simulink model "chutcalc_v2"  (R2019a)
settings: Solver=VariableStepDiscrete  StartTime=0.0  StopTime=10.0  RelTol=1e-3
undefined symbols (not defined in the file or in its folder): chutecalc_input
libraries: aerolibatmos2 x2
settings Model: Creator=onurd  LastModifiedBy=onurd

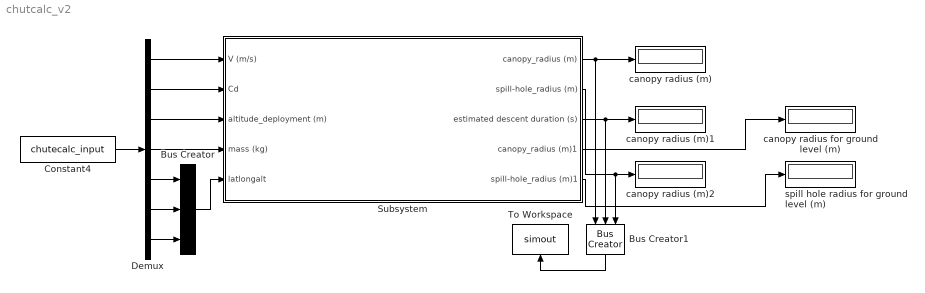
== system chutcalc_v2 ==
  " spill hole radius for ground level (m)" : Display
  Bus Creator : BusCreator  Inputs=3
  Bus Creator1 : BusCreator  Inputs=3
  Constant4 : Constant  Value=chutecalc_input
  Demux : Demux  Outputs=7
  Subsystem : Subsystem
  To Workspace : ToWorkspace  VariableName=simout  SampleTime=-1
      settings: MaxDataPoints=1  Save2DSignal=2-D array (concatenate along first dimension)
  canopy radius (m) : Display
  canopy radius (m)1 : Display
  canopy radius (m)2 : Display
  canopy radius for ground level (m) : Display
  wires:
  Subsystem/1(canopy_radius (m)) -> Bus Creator1/1, canopy radius (m)/1
  Constant4/1 -> Demux/1
  Demux/1 -> Subsystem/1(V (m/s))
  Demux/2 -> Subsystem/2(Cd)
  Demux/3 -> Subsystem/3(altitude_deployment (m))
  Demux/4 -> Subsystem/4(mass (kg))
  Demux/5 -> Bus Creator/1
  Demux/6 -> Bus Creator/2
  Demux/7 -> Bus Creator/3
  Bus Creator/1 -> Subsystem/5(latlongalt)
  Subsystem/2(spill-hole_radius (m)) -> canopy radius (m)1/1, Bus Creator1/2
  Subsystem/3(estimated descent duration (s)) -> canopy radius (m)2/1, Bus Creator1/3
  Bus Creator1/1 -> To Workspace/1
  Subsystem/4(canopy_radius (m)1) -> canopy radius for ground level (m)/1
  Subsystem/5(spill-hole_radius (m)1) -> " spill hole radius for ground level (m)"/1

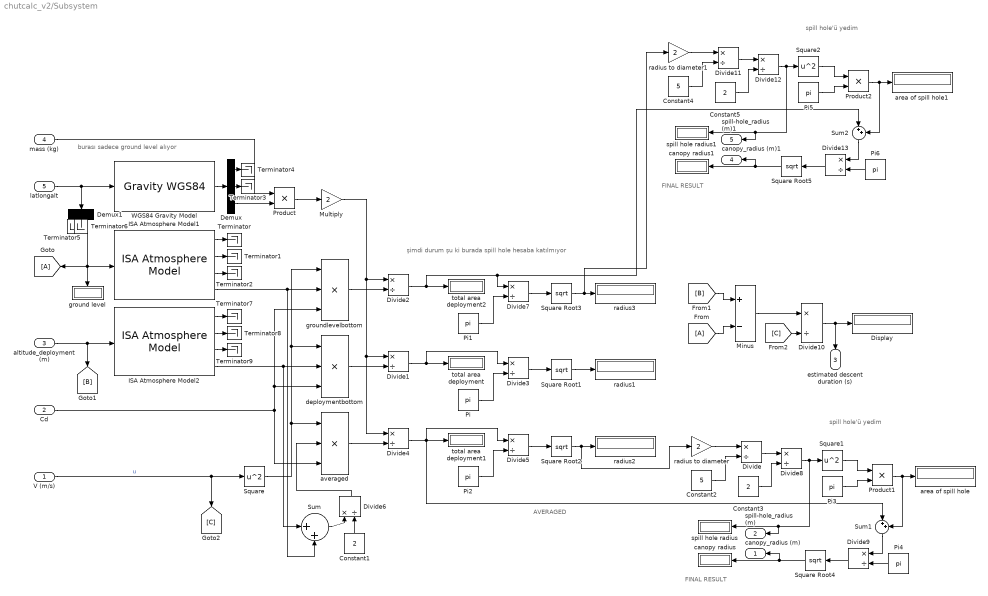
== system chutcalc_v2/Subsystem ==
  note: spill hole'ü yedim
  note: FINAL RESULT
  note: AVERAGED
  note: şimdi durum şu ki burada spill hole hesaba katılmıyor
  note: burası sadece ground level alıyor
  note: spill hole'ü yedim
  note: FINAL RESULT
  V (m/s) : Inport
  Cd : Inport  Port=2
  altitude_deployment (m) : Inport  Port=3
  mass (kg) : Inport  Port=4
  latlongalt : Inport  Port=5
  Constant1 : Constant  Value=2
  Constant2 : Constant  Value=5
  Constant3 : Constant  Value=2
  Constant4 : Constant  Value=5
  Constant5 : Constant  Value=2
  Demux : Demux  Outputs=3
  Demux1 : Demux  Outputs=3
  Display : Display
  Divide{,1..13} (14 alike) : Product  Inputs=*/
  ISA Atmosphere Model1 : aerolibatmos2/ISA Atmosphere Model  custom=off  g=9.80665  gamma=1.4  R=287.0531  L=0.0065  h_trop=11000  h_strat=20000  rho0=1.225  P0=101325  T0=288.15  h0=0
      settings: SourceProductName=Aerospace Blockset
  ISA Atmosphere Model2 : aerolibatmos2/ISA Atmosphere Model  custom=off  g=9.80665  gamma=1.4  R=287.0531  L=0.0065  h_trop=11000  h_strat=20000  rho0=1.225  P0=101325  T0=288.15  h0=0
      settings: SourceProductName=Aerospace Blockset
  Minus : Sum  Inputs=+-
  Multiply : Gain  Gain=2
  Pi{,1..6} (7 alike) : Constant  Value=pi  OutDataTypeStr=Inherit: Inherit via back propagation
  Product : Product
  Product1 : Product
  Product2 : Product
  Square : Math  Operator=square  SaturateOnIntegerOverflow=on
  Square Root{1..5} (5 alike) : Sqrt  SaturateOnIntegerOverflow=on
  Square1 : Math  Operator=square  SaturateOnIntegerOverflow=on
  Square2 : Math  Operator=square  SaturateOnIntegerOverflow=on
  Sum : Sum  Inputs=|++
  Sum1 : Sum  Inputs=|++
  Sum2 : Sum  Inputs=|++
  Terminator{,1..9} (10 alike) : Terminator
  "WGS84 Gravity Model  " : GravityWGS84  model=WGS84 Exact  month=May  day=9  year=2022
  area of spill hole : Display
  area of spill hole1 : Display
  averaged : Product  Inputs=3
  canopy radius : Display
  canopy radius1 : Display
  deploymentbottom : Product  Inputs=3
  ground level : Display
  groundlevelbottom : Product  Inputs=3
  radius to diameter : Gain  Gain=2
  radius to diameter1 : Gain  Gain=2
  radius1 : Display
  radius2 : Display
  radius3 : Display
  spill hole radius : Display
  spill hole radius1 : Display
  total area deployment : Display
  total area deployment1 : Display
  total area deployment2 : Display
  canopy_radius (m) : Outport
  spill-hole_radius (m) : Outport  Port=2
  estimated descent duration (s) : Outport  Port=3
  canopy_radius (m)1 : Outport  Port=4
  spill-hole_radius (m)1 : Outport  Port=5
  wires:
  Divide9/1 -> Square Root4/1
  Square/1 -> averaged/1, groundlevelbottom/1, deploymentbottom/1
  Product1/1 -> area of spill hole/1, Sum1/2
  ISA Atmosphere Model1/4 -> Sum/2, groundlevelbottom/2
  radius to diameter/1 -> Divide/1
  Divide3/1 -> Square Root1/1
  Divide1/1 -> Divide3/1, total area deployment/1
  Constant3/1 -> Divide8/2
  Cd/1 -> averaged/3, deploymentbottom/3, groundlevelbottom/3
  Divide4/1 -> Sum1/1, total area deployment1/1, Divide5/1
  Divide7/1 -> Square Root3/1
  Square Root1/1 -> radius1/1
  Demux1/3 -> ground level/1, [A], ISA Atmosphere Model1/1
  ISA Atmosphere Model2/4 -> deploymentbottom/2, Sum/1
  ISA Atmosphere Model2/3 -> Terminator9/1
  Divide6/1 -> averaged/2
  Constant1/1 -> Divide6/2
  Sum/1 -> Divide6/1
  ISA Atmosphere Model2/2 -> Terminator8/1
  Pi2/1 -> Divide5/2
  Pi3/1 -> Product1/2
  Constant2/1 -> Divide/2
  ISA Atmosphere Model1/3 -> Terminator2/1
  "WGS84 Gravity Model  "/1 -> Demux/1
  ISA Atmosphere Model1/1 -> Terminator/1
  V (m/s)/1 -> [C], Square/1  "u"
  Pi1/1 -> Divide7/2
  groundlevelbottom/1 -> Divide2/2
  mass (kg)/1 -> Product/1
  Pi/1 -> Divide3/2
  Divide5/1 -> Square Root2/1
  Square Root2/1 -> radius to diameter/1, radius2/1
  averaged/1 -> Divide4/2
  Product/1 -> Multiply/1
  Divide/1 -> Divide8/1
  Square Root4/1 -> canopy_radius (m)/1, canopy radius/1
  Multiply/1 -> Divide2/1, Divide4/1, Divide1/1
  Sum1/1 -> Divide9/1
  Demux/3 -> Product/2
  Divide8/1 -> spill-hole_radius (m)/1, spill hole radius/1, Square1/1
  Square1/1 -> Product1/1
  Pi4/1 -> Divide9/2
  latlongalt/1 -> "WGS84 Gravity Model  "/1, Demux1/1
  altitude_deployment (m)/1 -> [B], ISA Atmosphere Model2/1
  deploymentbottom/1 -> Divide1/2
  ISA Atmosphere Model2/1 -> Terminator7/1
  ISA Atmosphere Model1/2 -> Terminator1/1
  Minus/1 -> Divide10/1
  [B] -> Minus/1
  [A] -> Minus/2
  [C] -> Divide10/2
  Divide10/1 -> estimated descent duration (s)/1, Display/1
  Demux1/1 -> Terminator5/1
  Demux1/2 -> Terminator6/1
  Demux/2 -> Terminator3/1
  Demux/1 -> Terminator4/1
  Pi6/1 -> Divide13/2
  Square2/1 -> Product2/1
  Divide12/1 -> Square2/1, spill hole radius1/1, spill-hole_radius (m)1/1
  Sum2/1 -> Divide13/1
  Square Root5/1 -> canopy radius1/1, canopy_radius (m)1/1
  Divide11/1 -> Divide12/1
  Square Root3/1 -> radius to diameter1/1, radius3/1
  Constant4/1 -> Divide11/2
  Pi5/1 -> Product2/2
  Divide2/1 -> Sum2/1, Divide7/1, total area deployment2/1
  Constant5/1 -> Divide12/2
  radius to diameter1/1 -> Divide11/1
  Product2/1 -> Sum2/2, area of spill hole1/1
  Divide13/1 -> Square Root5/1
